simulink model "z1"  (R2017b)
settings: Solver=FixedStepDiscrete  StartTime=0.0  StopTime=0.0  RelTol=1e-3
libraries: CPOiS_SourcesSinks x12, CPOiS_DataManipulation x6
settings Model: Creator=alis  LastModifiedBy=alis

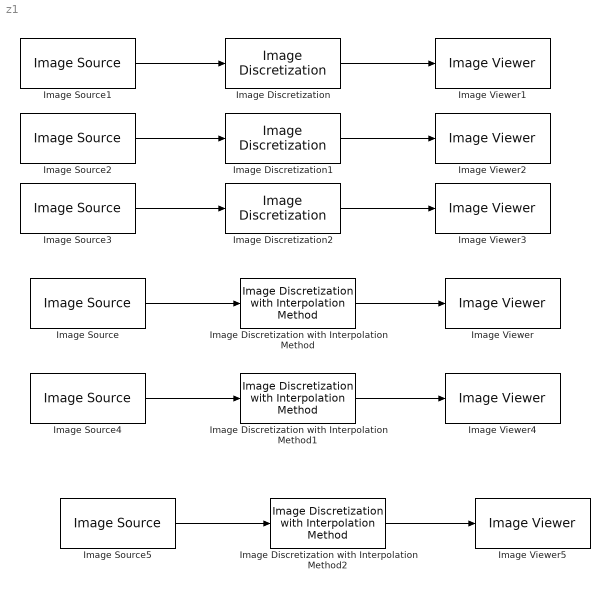
== system z1 ==
  Image Discretization : CPOiS_DataManipulation/Image Discretization  factor=2
      settings: SourceProductName=CPOiS - Digital image and signal processing
  Image Discretization with Interpolation Method : CPOiS_DataManipulation/Image Discretization with Interpolation Method  factor=4  method=nearest
      settings: SourceProductName=CPOiS - Digital image and signal processing
  Image Discretization with Interpolation Method1 : CPOiS_DataManipulation/Image Discretization with Interpolation Method  factor=4  method=bilinear
      settings: SourceProductName=CPOiS - Digital image and signal processing
  Image Discretization with Interpolation Method2 : CPOiS_DataManipulation/Image Discretization with Interpolation Method  factor=4  method=bicubic
      settings: SourceProductName=CPOiS - Digital image and signal processing
  Image Discretization1 : CPOiS_DataManipulation/Image Discretization  factor=4
      settings: SourceProductName=CPOiS - Digital image and signal processing
  Image Discretization2 : CPOiS_DataManipulation/Image Discretization  factor=8
      settings: SourceProductName=CPOiS - Digital image and signal processing
  Image Source{,1..5} (6 alike) : CPOiS_SourcesSinks/Image Source  FileSelection=gull.png
      settings: SourceProductName=CPOiS - Digital image and signal processing
  Image Viewer{,1..5} (6 alike) : CPOiS_SourcesSinks/Image Viewer
      settings: SourceProductName=CPOiS - Digital image and signal processing
  wires:
  Image Source1/1 -> Image Discretization/1
  Image Discretization/1 -> Image Viewer1/1
  Image Source/1 -> Image Discretization with Interpolation Method/1
  Image Discretization with Interpolation Method/1 -> Image Viewer/1
  Image Source2/1 -> Image Discretization1/1
  Image Discretization1/1 -> Image Viewer2/1
  Image Source3/1 -> Image Discretization2/1
  Image Discretization2/1 -> Image Viewer3/1
  Image Discretization with Interpolation Method1/1 -> Image Viewer4/1
  Image Source4/1 -> Image Discretization with Interpolation Method1/1
  Image Discretization with Interpolation Method2/1 -> Image Viewer5/1
  Image Source5/1 -> Image Discretization with Interpolation Method2/1
